simulink model "comparison_ctrl_2022_03_08"  (R2021b)
settings: Solver=VariableStepAuto  StartTime=0.0  StopTime=simlegth  RelTol=1e-3
values from neighbouring files (symbols this model uses):
  Ad = [cos(w*ts) sin(w*ts)/w; -w*sin(w*ts) cos(w*ts)]    [pres_ctrl_design.m]    (also in resonant_PI.m = [cos(w*Ts) sin(w*Ts)/w; -w*sin(w*Ts) cos(w*Ts)])
  Bd = [(1-cos(w*ts))/w^2 sin(w*ts)/w]'    [pres_ctrl_design.m]    (also in resonant_PI.m = [(1-cos(w*Ts))/w^2 sin(w*Ts)/w]')
  C = [0 1]    [pres_ctrl_design.m]    (also in resonant_PI.m)
  ki = 18    [pres_ctrl_design.m]    (also in resonant_PI.m = 8)
  kp = 0.5    [pres_ctrl_design.m]    (also in resonant_PI.m = 0.1)
  s = tf('s')    [pres_ctrl_design.m]    (also in resonant_PI.m)
  Tc = ts/10    (= 0.0001)    [pres_ctrl_design.m]    (also in resonant_PI.m = 1e-05)
  Ts = 1e-4    (= 0.0001)    [resonant_PI.m]
  w = 2*pi*50    (= 314.159265359)    [pres_ctrl_design.m]    (also in resonant_PI.m)
libraries: cstblocks x9
settings Model: Creator=dabagnara  LastModifiedBy=dabagnara
settings SolverCC: AlgebraicLoopSolver=TrustRegion
settings DataIOCC: ReturnWorkspaceOutputs=off
settings DebuggingCC: SFMachineParentedDataDiag=warning

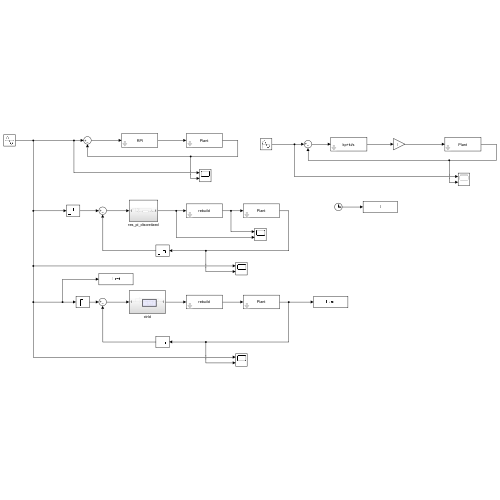
[thumbnail: Simulink's stored preview of the top-level diagram]
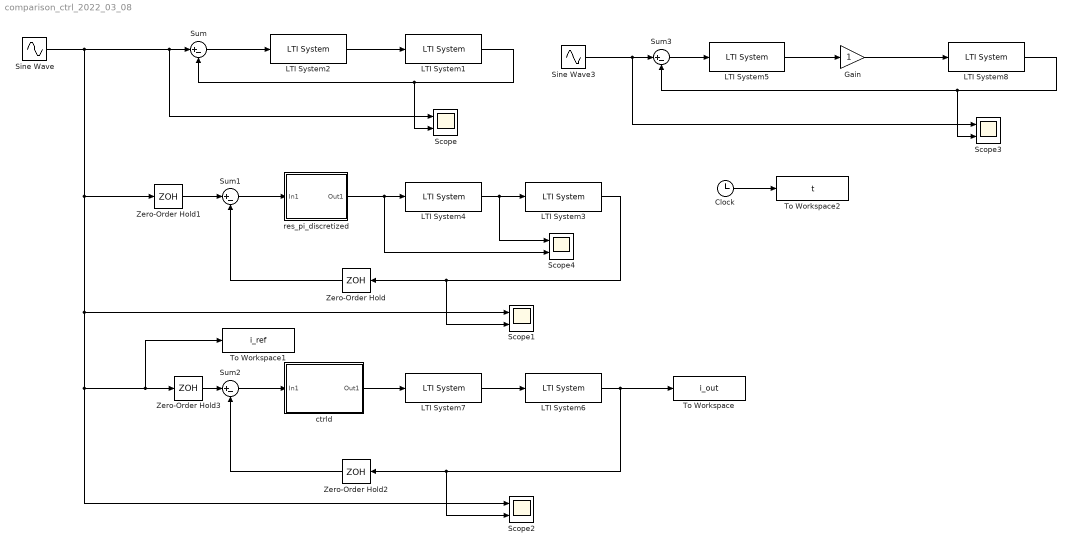
== system comparison_ctrl_2022_03_08 ==
  Clock : Clock
  Gain : Gain
  LTI System{1,3,6,8} (4 alike) : cstblocks/LTI System  sys=Plant  IC=[]
  LTI System2 : cstblocks/LTI System  sys=RPI  IC=[0]
  LTI System4 : cstblocks/LTI System  sys=rebuild  IC=[0]
  LTI System5 : cstblocks/LTI System  sys=kp+ki/s  IC=[]
  LTI System7 : cstblocks/LTI System  sys=rebuild  IC=[0]
  Scope{,1..4} (5 alike) : Scope  NumInputPorts=2
  Sine Wave : Sin  Frequency=w  SampleTime=0
  Sine Wave3 : Sin  Frequency=w  SampleTime=0
  Sum{,1..3} (4 alike) : Sum  Inputs=|+-
  To Workspace : ToWorkspace  VariableName=i_out  SampleTime=Tc
  To Workspace1 : ToWorkspace  VariableName=i_ref  SampleTime=Tc
  To Workspace2 : ToWorkspace  VariableName=t  SampleTime=Tc
  Zero-Order Hold{,1..3} (4 alike) : ZeroOrderHold  SampleTime=Ts
  ctrld : Subsystem
  res_pi_discretized : Subsystem
  wires:
  Sum/1 -> LTI System2/1
  LTI System2/1 -> LTI System1/1
  LTI System1/1 -> Scope/2, Sum/2
  Sum1/1 -> res_pi_discretized/1(In1)
  Zero-Order Hold/1 -> Sum1/2
  Zero-Order Hold1/1 -> Sum1/1
  res_pi_discretized/1(Out1) -> Scope4/2, LTI System4/1
  LTI System4/1 -> Scope4/1, LTI System3/1
  LTI System7/1 -> LTI System6/1
  Zero-Order Hold3/1 -> Sum2/1
  Zero-Order Hold2/1 -> Sum2/2
  Sine Wave/1 -> Scope/1, Sum/1, Zero-Order Hold1/1, Scope1/1, To Workspace1/1, Zero-Order Hold3/1, Scope2/1
  LTI System6/1 -> Scope2/2, Zero-Order Hold2/1, To Workspace/1
  Sum2/1 -> ctrld/1(In1)
  ctrld/1(Out1) -> LTI System7/1
  Sine Wave3/1 -> Sum3/1, Scope3/1
  LTI System8/1 -> Sum3/2, Scope3/2
  LTI System5/1 -> Gain/1
  Sum3/1 -> LTI System5/1
  Gain/1 -> LTI System8/1
  LTI System3/1 -> Zero-Order Hold/1, Scope1/2
  Clock/1 -> To Workspace2/1

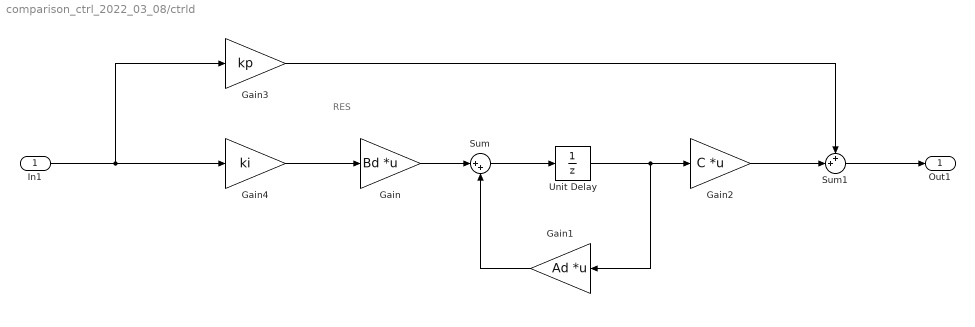
== system comparison_ctrl_2022_03_08/ctrld ==
  note: RES
  In1 : Inport
  Gain : Gain  Gain=Bd  Multiplication=Matrix(K*u)
  Gain1 : Gain  Gain=Ad  Multiplication=Matrix(K*u)
  Gain2 : Gain  Gain=C  Multiplication=Matrix(K*u)
  Gain3 : Gain  Gain=kp
  Gain4 : Gain  Gain=ki
  Sum : Sum  Inputs=|++
  Sum1 : Sum  Inputs=++|
  Unit Delay : UnitDelay  SampleTime=Ts  HasFrameUpgradeWarning=on
  Out1 : Outport
  wires:
  In1/1 -> Gain4/1, Gain3/1
  Sum/1 -> Unit Delay/1
  Gain/1 -> Sum/1
  Gain1/1 -> Sum/2
  Unit Delay/1 -> Gain2/1, Gain1/1
  Gain4/1 -> Gain/1
  Gain2/1 -> Sum1/2
  Sum1/1 -> Out1/1
  Gain3/1 -> Sum1/1

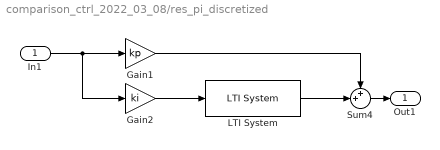
== system comparison_ctrl_2022_03_08/res_pi_discretized ==
  In1 : Inport
  Gain1 : Gain  Gain=kp
  Gain2 : Gain  Gain=ki
  LTI System : cstblocks/LTI System  sys=RESd3  IC=[]
  Sum4 : Sum  Inputs=++|
  Out1 : Outport
  wires:
  In1/1 -> Gain2/1, Gain1/1
  LTI System/1 -> Sum4/2
  Gain1/1 -> Sum4/1
  Sum4/1 -> Out1/1
  Gain2/1 -> LTI System/1
